simulink model "blackbanana_kincon"  (R2022b)
settings: Solver=VariableStepAuto  StartTime=0.0  StopTime=20  RelTol=1e-3
libraries: VACLib x4
settings Model: Creator=KarlO  LastModifiedBy=KarlO

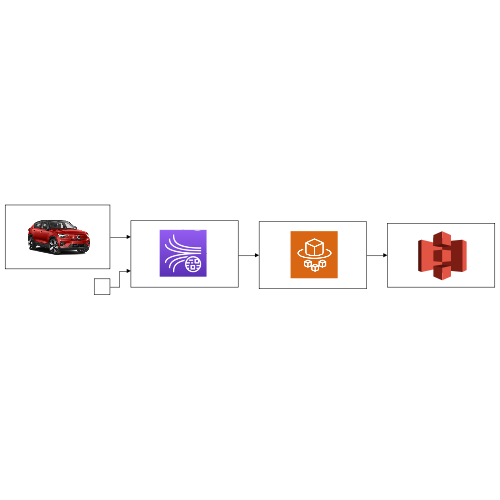
[thumbnail: Simulink's stored preview of the top-level diagram]
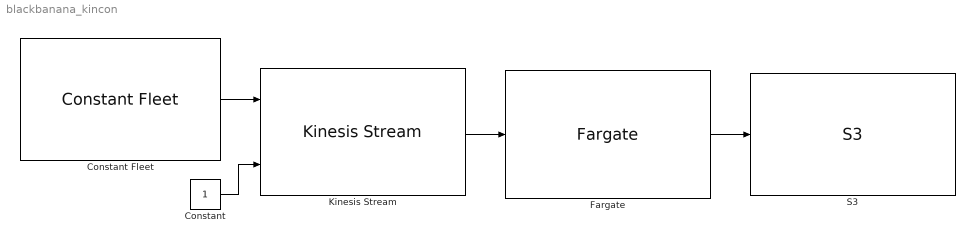
== system blackbanana_kincon ==
  Constant : Constant
  Constant Fleet : VACLib/Vehicle Components/Constant Fleet  SystemSampleTime=-1  VariantActivationTime=update diagram  Latency=0  AutoFrameSizeCalculation=off
      settings: SourceProductName=Volvo Architechture Components
  Fargate : VACLib/AWS Components/Fargate  SystemSampleTime=-1  VariantActivationTime=update diagram  Latency=0  AutoFrameSizeCalculation=off
      settings: SourceProductName=Volvo Architechture Components
  Kinesis Stream : VACLib/AWS Components/Kinesis Stream  SystemSampleTime=-1  VariantActivationTime=update diagram  Latency=0  AutoFrameSizeCalculation=off
      settings: SourceProductName=Volvo Architechture Components
  S3 : VACLib/AWS Components/S3  SystemSampleTime=-1  VariantActivationTime=update diagram  Latency=0  AutoFrameSizeCalculation=off
      settings: SourceProductName=Volvo Architechture Components
  wires:
  Constant Fleet/1 -> Kinesis Stream/1
  Fargate/1 -> S3/1
  Kinesis Stream/1 -> Fargate/1
  Constant/1 -> Kinesis Stream/2
